simulink model "MV_szabalzo_simulink"  (R2021a)
settings: Solver=VariableStepAuto  StartTime=0.0  StopTime=10.0  RelTol=1e-3
values from neighbouring files (symbols this model uses):
  A = [1 -1.5 0.54]    [MV_szab_nem_adaptiv.m]
  B = [2 -1.8]    [MV_szab_nem_adaptiv.m]
  C = [1 0.2 -.48]    [MV_szab_nem_adaptiv.m]
undefined symbols (not defined in the file or in its folder): F, G
settings Model: Creator=Krisz  LastModifiedBy=Krisz

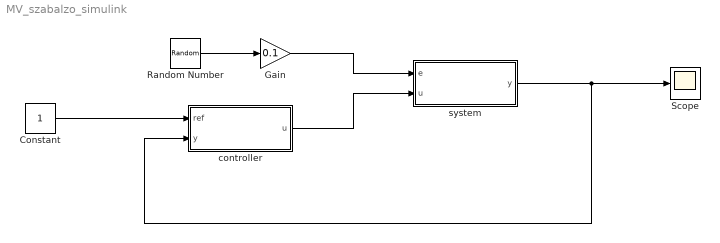
== system MV_szabalzo_simulink ==
  Constant : Constant
  Gain : Gain  Gain=0.1
  Random Number : RandomNumber  Variance=0.01  SampleTime=0.1
  Scope : Scope
  controller : Subsystem  mask{A=A, B=B, C=C, F=F, G=G}
  system : Subsystem  mask{A=A, B=B, C=C}
  wires:
  controller/1(u) -> system/2(u)
  system/1(y) -> controller/2(y), Scope/1
  Random Number/1 -> Gain/1
  Gain/1 -> system/1(e)
  Constant/1 -> controller/1(ref)

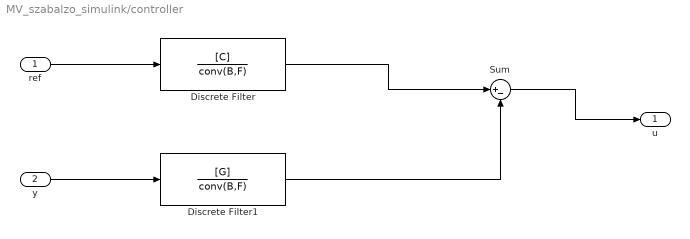
== system MV_szabalzo_simulink/controller ==
  ref : Inport
  y : Inport  Port=2
  Discrete Filter : DiscreteFilter  Numerator=[C]  Denominator=conv(B,F)
  Discrete Filter1 : DiscreteFilter  Numerator=[G]  Denominator=conv(B,F)
  Sum : Sum  Inputs=|+-
  u : Outport
  wires:
  Discrete Filter/1 -> Sum/1
  Discrete Filter1/1 -> Sum/2
  ref/1 -> Discrete Filter/1
  y/1 -> Discrete Filter1/1
  Sum/1 -> u/1

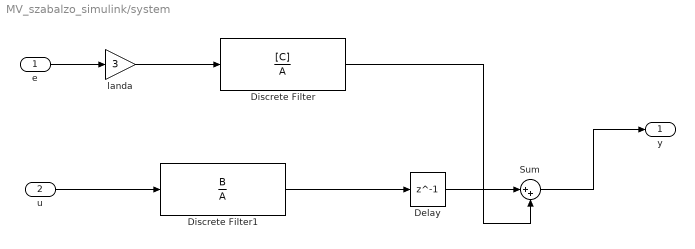
== system MV_szabalzo_simulink/system ==
  e : Inport
  u : Inport  Port=2
  Delay : Delay  DelayLength=1  InitialCondition=0
  Discrete Filter : DiscreteFilter  Numerator=[C]  Denominator=A
  Discrete Filter1 : DiscreteFilter  Numerator=B  Denominator=A
  Sum : Sum  Inputs=|++
  landa : Gain  Gain=3
  y : Outport
  wires:
  Discrete Filter1/1 -> Delay/1
  Delay/1 -> Sum/1
  Discrete Filter/1 -> Sum/2
  landa/1 -> Discrete Filter/1
  u/1 -> Discrete Filter1/1
  e/1 -> landa/1
  Sum/1 -> y/1
